simulink model "soccerbot"  (R2017b)
settings: Solver=FixedStepDiscrete  StartTime=0.0  StopTime=inf  FixedStep=0.01  RelTol=1e-3
PreLoadFcn:
  | clear;
  | 
  | % Sample times
  | sampleTime = 0.2;
  | 
  | % Control parameters
  | ctrlParam1 = 2;
  | ctrlParam2 = 3.5;
  | 
  | loadIpAddresses;
InitFcn:
  | loadFixedTrajectories;
model workspace (MAT data in the model file):
  SL_ROS_VariableLengthArrays_MaxSizes.CommonInfo.ArrayTruncateAction = 'EmitWarning'
  SL_ROS_VariableLengthArrays_MaxSizes.MsgTypeMap = containers.Map
  SL_ROS_VariableLengthArrays_MaxSizes.MsgTypeMap.serialization.keys = {'sensor_msgs/Image'}
  SL_ROS_VariableLengthArrays_MaxSizes.MsgTypeMap.serialization.values{1}(1).PropertyName = 'Data'
  SL_ROS_VariableLengthArrays_MaxSizes.MsgTypeMap.serialization.values{1}(1).DataType = 'uint8'
  SL_ROS_VariableLengthArrays_MaxSizes.MsgTypeMap.serialization.values{1}(1).MaxLength = 230400
  SL_ROS_VariableLengthArrays_MaxSizes.MsgTypeMap.serialization.values{1}(2).PropertyName = 'Encoding'
  SL_ROS_VariableLengthArrays_MaxSizes.MsgTypeMap.serialization.values{1}(2).DataType = 'uint8'
  SL_ROS_VariableLengthArrays_MaxSizes.MsgTypeMap.serialization.values{1}(2).MaxLength = 128
  SL_ROS_VariableLengthArrays_MaxSizes.MsgTypeMap.serialization.uniformity = 0
  SL_ROS_VariableLengthArrays_MaxSizes.MsgTypeMap.serialization.keyType = 'char'
  SL_ROS_VariableLengthArrays_MaxSizes.MsgTypeMap.serialization.valueType = 'any'
  ctrlParam1 = 1
  ctrlParam2 = 1.5
  sampleTime = 0.01
undefined symbols (not defined in the file): customState, getUpBackTraj, getUpFrontTraj, resting, walkTraj
libraries: simulink x54, robotlib x4, commblkintrlv2 x2, visionsinks x1
settings Model: Creator=scastro  LastModifiedBy=vuwij
settings OptimizationCC: PassReuseOutputArgsThreshold=0  EfficientMapNaN2IntZero=off  MaxStackSize=64
settings DebuggingCC: ParameterTunabilityLossMsg=error
settings HardwareCC: ProdBitPerPointer=32  ProdBitPerSizeT=32  ProdBitPerPtrDiffT=32  ProdLargestAtomicFloat=None  ProdIntDivRoundTo=Undefined  ProdEndianess=Unspecified  ProdWordSize=32  ProdHWDeviceType=Generic->Unspecified (assume 32-bit Generic)  TargetBitPerLong=64  TargetBitPerPointer=64  TargetBitPerSizeT=64  TargetBitPerPtrDiffT=64  TargetLongLongMode=on  TargetIntDivRoundTo=Zero  TargetEndianess=LittleEndian  TargetWordSize=64  TargetHWDeviceType=MATLAB Host  ProdEqTarget=off
settings SFSimCC: MATLABDynamicMemAlloc=off
settings RTWCC: TargetLang=C++
settings CodeAppCC: MaxIdLength=128
settings GRTTargetCC: TargetLangStandard=C89/C90 (ANSI)  CombineOutputUpdateFcns=off  GRTInterface=on

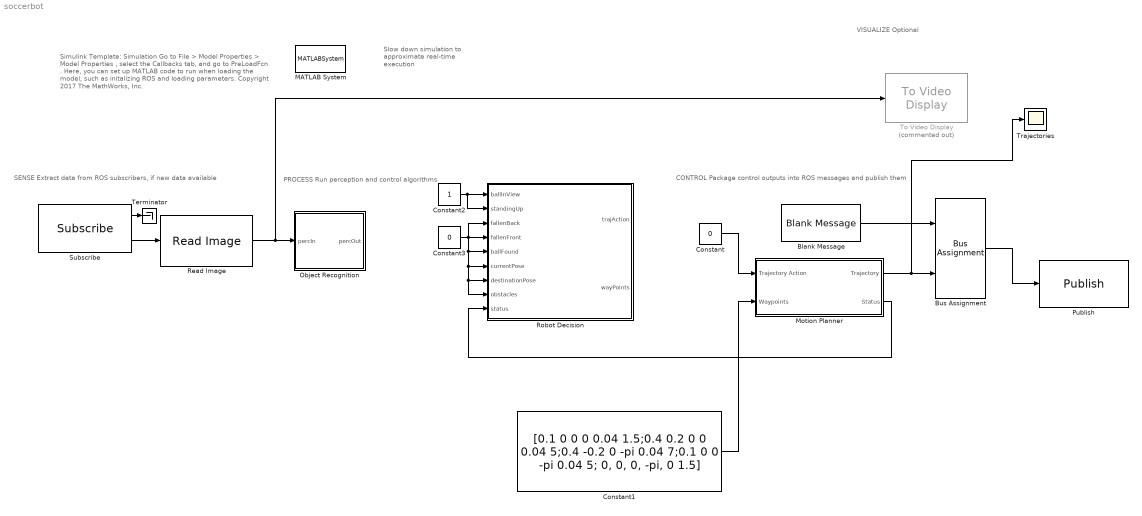
== system soccerbot ==
  note: Simulink Template: Simulation
      |
      | Go to File > Model Properties > Model Properties , select the Callbacks tab, and go to PreLoadFcn .
      |
      | Here, you can set up MATLAB code to run when loading the model, such as initalizing ROS and loading parameters.
      |
      | Copyright 2017 The MathWorks, Inc.
  note: Slow down simulation to approximate real-time execution
  note: PROCESS
      | Run perception and control algorithms
  note: SENSE
      | Extract data from ROS subscribers, if new data available
  note: VISUALIZE
      | Optional
  note: CONTROL
      | Package control outputs into ROS messages and publish them
  Blank Message : robotlib/Blank Message  SourceLibraryInfo=This block requires Robotics System Toolbox  messageType=soccer_msgs/RobotGoal  SampleTime=inf
      settings: SourceProductBaseCode=RO
  Bus Assignment : BusAssignment  AssignedSignals=Trajectories
  Constant : Constant  Value=0
  Constant1 : Constant  Value=[0.1 0 0 0 0.04 1.5;0.4 0.2 0 0 0.04 5;0.4 -0.2 0 -pi 0.04 7;0.1 0 0 -pi 0.04 5; 0, 0, 0, -pi, 0 1.5]  VectorParams1D=off
  Constant2 : Constant
  Constant3 : Constant  Value=0
  MATLAB System : MATLABSystem  System=ExampleHelperSimulationRateControl  SampleTime=sampleTime
      mask Type: ExampleHelperSimulationRateControl
      mask Display: disp('Rate Control');
  Motion Planner : Subsystem
  Object Recognition : Subsystem
  Publish : robotlib/Publish  SourceLibraryInfo=This block requires Robotics System Toolbox  topicSource=Select from ROS network  topic=/robotGoal  messageType=soccer_msgs/RobotGoal  messageQueueLength=1
      settings: SourceProductBaseCode=RO
  Read Image : robotlib/Read Image  SourceLibraryInfo=This block requires Robotics System Toolbox  MaximumImageSize=[240, 320]  ImageEncoding=rgb8  ShowAlphaOutput=off  ShowErrorCodeOutput=off  VariableSizeOutputs=off
      settings: SourceProductName=Robotics System Toolbox  SourceProductBaseCode=RO
  Robot Decision : Stateflow chart  TreatAsAtomicUnit=on
  Subscribe : robotlib/Subscribe  SourceLibraryInfo=This block requires Robotics System Toolbox  topicSource=Select from ROS network  topic=/soccerbot/camera1/image_raw  messageType=sensor_msgs/Image  sampleTime=-1  messageQueueLength=1
      settings: SourceProductBaseCode=RO
  Terminator : Terminator
  To Video Display : visionsinks/To Video Display  Commented=on  windowSizeMode=Normal  openAtMdlStart=on  fullScreen=off  videoWindowX=275  videoWindowY=548  saveWindowSize=off  videoWindowWidth=320  videoWindowHeight=240  inputColorFormat=RGB  inputType=Obsolete  imagePorts=One multidimensional signal  OutputDevice=On-screen video monitor  dataOrg=Column-major  isWindowOpen=off
      settings: SourceProductName=Computer Vision System Toolbox
  Trajectories : Scope
  wires:
  Read Image/1 -> To Video Display/1, Object Recognition/1(percIn)
  Subscribe/2 -> Read Image/1
  Subscribe/1 -> Terminator/1
  Motion Planner/1(Trajectory) -> Trajectories/1, Bus Assignment/2
  Bus Assignment/1 -> Publish/1
  Blank Message/1 -> Bus Assignment/1
  Constant1/1 -> Motion Planner/2(Waypoints)
  Constant/1 -> Motion Planner/1(Trajectory Action)
  Constant2/1 -> Robot Decision/2(standingUp), Robot Decision/1(ballInView)
  Constant3/1 -> Robot Decision/3(fallenBack), Robot Decision/8(obstacles), Robot Decision/7(destinationPose), Robot Decision/6(currentPose), Robot Decision/5(ballFound), Robot Decision/4(fallenFront)
  Motion Planner/2(Status) -> Robot Decision/9(status)

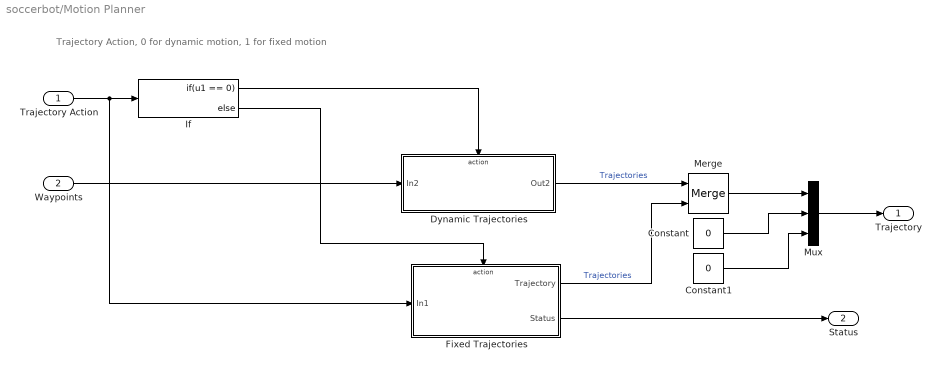
== system soccerbot/Motion Planner ==
  note: Trajectory Action, 0 for dynamic motion, 1 for fixed motion
  Trajectory Action : Inport
  Waypoints : Inport  Port=2
  Constant : Constant  Value=0  OutDataTypeStr=single
  Constant1 : Constant  Value=0  OutDataTypeStr=single
  Dynamic Trajectories : Subsystem  TreatAsAtomicUnit=on
  Fixed Trajectories : Subsystem  TreatAsAtomicUnit=on
  If : If  IfExpression=u1 == 0
  Merge : Merge
  Mux : Mux  Inputs=3
  Trajectory : Outport
  Status : Outport  Port=2
  wires:
  Dynamic Trajectories/1(Out2) -> Merge/1  "Trajectories"
  If/1 -> Dynamic Trajectories/Action
  Trajectory Action/1 -> Fixed Trajectories/1(In1), If/1
  Fixed Trajectories/1(Trajectory) -> Merge/2  "Trajectories"
  If/2 -> Fixed Trajectories/Action
  Waypoints/1 -> Dynamic Trajectories/1(In2)
  Fixed Trajectories/2(Status) -> Status/1
  Merge/1 -> Mux/1
  Mux/1 -> Trajectory/1
  Constant/1 -> Mux/2
  Constant1/1 -> Mux/3

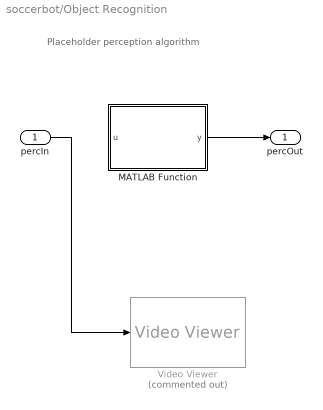
== system soccerbot/Object Recognition ==
  note: Placeholder perception algorithm
  percIn : Inport
  MATLAB Function : MATLAB Function  TreatAsAtomicUnit=on
  Video Viewer : VideoViewer  Commented=on  FigPos=[511 723 604 426]
  percOut : Outport
  wires:
  percIn/1 -> Video Viewer/1
  MATLAB Function/1(y) -> percOut/1

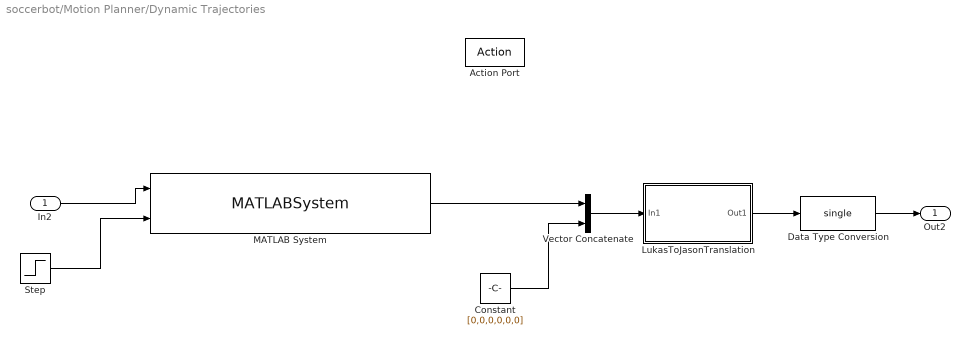
== system soccerbot/Motion Planner/Dynamic Trajectories ==
  In2 : Inport
  Action Port : ActionPort  ActionType=then
  Constant : Constant  Value=[0,0,0,0,0,0]
  Data Type Conversion : DataTypeConversion  OutDataTypeStr=single
  LukasToJasonTranslation : Subsystem  TreatAsAtomicUnit=on
  MATLAB System : MATLABSystem  System=BipedalRobotSystemObject  SimulateUsing=Interpreted execution
      mask Type: BipedalRobotSystemObject
      mask Display:
      | disp('BipedalRobotSystemObject');
      | port_label('input',1,'waypoints');
      | port_label('input',2,'trigger');
      | port_label('output',1,'trajectories');
  Step : Step  Time=3  SampleTime=0
  Vector Concatenate : Concatenate
  Out2 : Outport
  wires:
  In2/1 -> MATLAB System/1
  Constant/1 -> Vector Concatenate/2
  Vector Concatenate/1 -> LukasToJasonTranslation/1(In1)
  Step/1 -> MATLAB System/2
  MATLAB System/1 -> Vector Concatenate/1
  LukasToJasonTranslation/1(Out1) -> Data Type Conversion/1
  Data Type Conversion/1 -> Out2/1

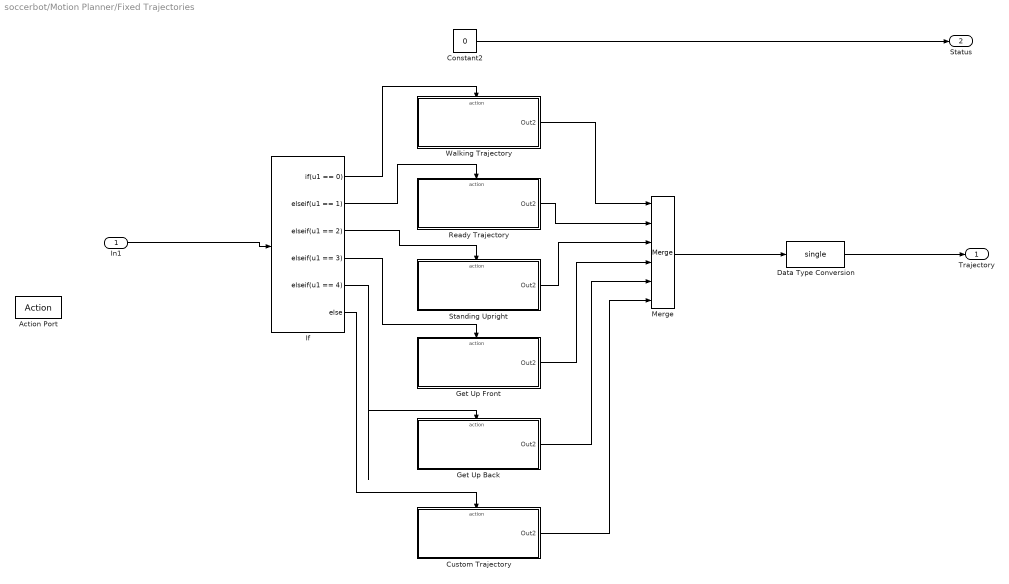
== system soccerbot/Motion Planner/Fixed Trajectories ==
  In1 : Inport
  Action Port : ActionPort  ActionType=else
  Constant2 : Constant  Value=0
  "Custom Trajectory " : Subsystem  TreatAsAtomicUnit=on
  Data Type Conversion : DataTypeConversion  OutDataTypeStr=single
  Get Up Back : Subsystem  TreatAsAtomicUnit=on
  Get Up Front : Subsystem  TreatAsAtomicUnit=on
  If : If  IfExpression=u1 == 0  ElseIfExpressions=u1 == 1, u1 == 2, u1 == 3, u1 == 4
  Merge : Merge  Inputs=6
  Ready Trajectory : Subsystem  TreatAsAtomicUnit=on
  Standing Upright : Subsystem  TreatAsAtomicUnit=on
  Walking Trajectory : Subsystem  TreatAsAtomicUnit=on
  Trajectory : Outport
  Status : Outport  Port=2
  wires:
  Standing Upright/1(Out2) -> Merge/3
  Get Up Back/1(Out2) -> Merge/5
  If/4 -> Get Up Front/Action
  If/1 -> Walking Trajectory/Action
  Walking Trajectory/1(Out2) -> Merge/1
  Data Type Conversion/1 -> Trajectory/1
  Ready Trajectory/1(Out2) -> Merge/2
  Merge/1 -> Data Type Conversion/1
  If/6 -> "Custom Trajectory "/Action
  In1/1 -> If/1
  "Custom Trajectory "/1(Out2) -> Merge/6
  If/5 -> Get Up Back/Action
  If/3 -> Standing Upright/Action
  Constant2/1 -> Status/1
  Get Up Front/1(Out2) -> Merge/4
  If/2 -> Ready Trajectory/Action

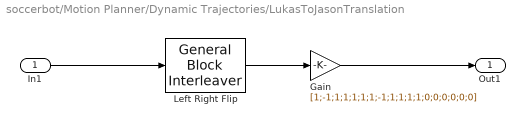
== system soccerbot/Motion Planner/Dynamic Trajectories/LukasToJasonTranslation ==
  In1 : Inport
  Gain : Gain  Gain=[1;-1;1;1;1;1;1;-1;1;1;1;1;0;0;0;0;0;0]
  Left Right Flip : commblkintrlv2/General Block Interleaver  permutationVectorSource=Dialog  elements=[7;8;9;10;11;12;1;2;3;4;5;6;13;14;15;16;17;18]
      settings: SourceProductName=Communications System Toolbox  SourceProductBaseCode=CM
  Out1 : Outport
  wires:
  In1/1 -> Left Right Flip/1
  Gain/1 -> Out1/1
  Left Right Flip/1 -> Gain/1

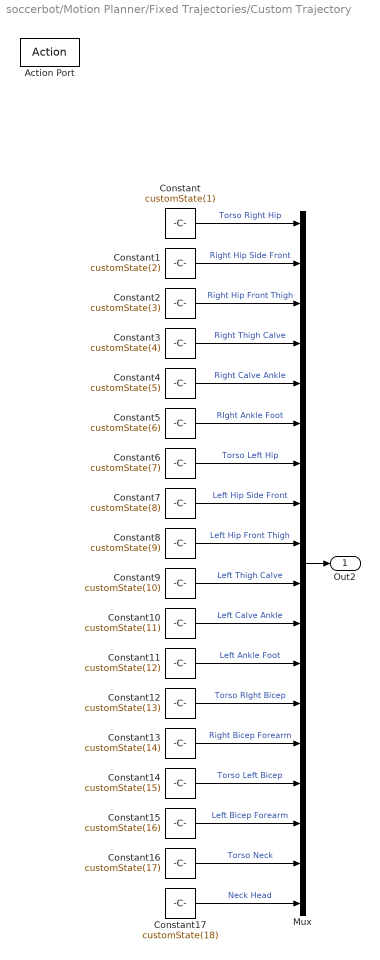
== system soccerbot/Motion Planner/Fixed Trajectories/Custom Trajectory  ==
  Action Port : ActionPort  ActionType=else
  Constant : Constant  Value=customState(1)
  Constant1 : Constant  Value=customState(2)
  Constant10 : Constant  Value=customState(11)
  Constant11 : Constant  Value=customState(12)
  Constant12 : Constant  Value=customState(13)
  Constant13 : Constant  Value=customState(14)
  Constant14 : Constant  Value=customState(15)
  Constant15 : Constant  Value=customState(16)
  Constant16 : Constant  Value=customState(17)
  Constant17 : Constant  Value=customState(18)
  Constant2 : Constant  Value=customState(3)
  Constant3 : Constant  Value=customState(4)
  Constant4 : Constant  Value=customState(5)
  Constant5 : Constant  Value=customState(6)
  Constant6 : Constant  Value=customState(7)
  Constant7 : Constant  Value=customState(8)
  Constant8 : Constant  Value=customState(9)
  Constant9 : Constant  Value=customState(10)
  Mux : Mux  Inputs=18
  Out2 : Outport
  wires:
  Constant3/1 -> Mux/4  "Right Thigh Calve"
  Constant12/1 -> Mux/13  "Torso RIght Bicep"
  Constant8/1 -> Mux/9  "Left Hip Front Thigh"
  Constant1/1 -> Mux/2  "Right Hip Side Front"
  Constant14/1 -> Mux/15  "Torso Left Bicep"
  Constant9/1 -> Mux/10  "Left Thigh Calve"
  Constant17/1 -> Mux/18  "Neck Head"
  Constant11/1 -> Mux/12  "Left Ankle Foot"
  Constant16/1 -> Mux/17  "Torso Neck"
  Constant10/1 -> Mux/11  "Left Calve Ankle"
  Constant15/1 -> Mux/16  "Left Bicep Forearm"
  Constant13/1 -> Mux/14  "Right Bicep Forearm"
  Constant/1 -> Mux/1  "Torso Right Hip"
  Mux/1 -> Out2/1
  Constant7/1 -> Mux/8  "Left Hip Side Front"
  Constant2/1 -> Mux/3  "Right Hip Front Thigh"
  Constant6/1 -> Mux/7  "Torso Left Hip"
  Constant4/1 -> Mux/5  "Right Calve Ankle"
  Constant5/1 -> Mux/6  "RIght Ankle Foot"

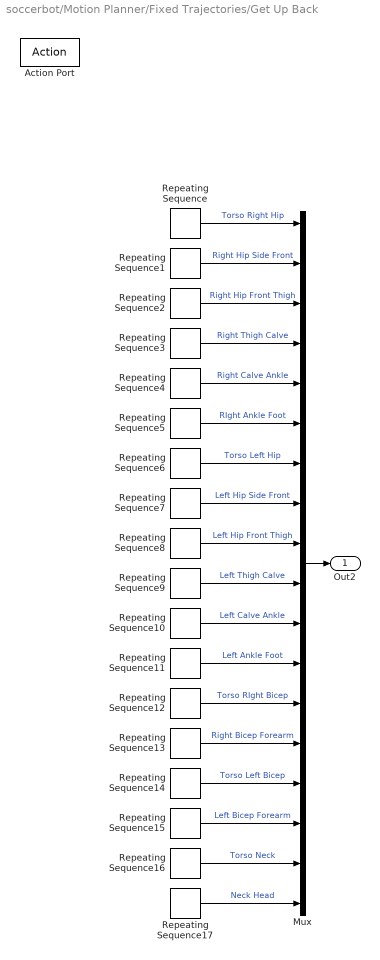
== system soccerbot/Motion Planner/Fixed Trajectories/Get Up Back ==
  Action Port : ActionPort  ActionType=elseif
  Mux : Mux  Inputs=18
  Repeating Sequence : simulink/Sources/Repeating Sequence  rep_seq_t=getUpBackTrajTime  rep_seq_y=getUpBackTraj(:,1)
  Repeating Sequence1 : simulink/Sources/Repeating Sequence  rep_seq_t=getUpBackTrajTime  rep_seq_y=getUpBackTraj(:,2)
  Repeating Sequence10 : simulink/Sources/Repeating Sequence  rep_seq_t=getUpBackTrajTime  rep_seq_y=getUpBackTraj(:,11)
  Repeating Sequence11 : simulink/Sources/Repeating Sequence  rep_seq_t=getUpBackTrajTime  rep_seq_y=getUpBackTraj(:,12)
  Repeating Sequence12 : simulink/Sources/Repeating Sequence  rep_seq_t=getUpBackTrajTime  rep_seq_y=getUpBackTraj(:,13)
  Repeating Sequence13 : simulink/Sources/Repeating Sequence  rep_seq_t=getUpBackTrajTime  rep_seq_y=getUpBackTraj(:,14)
  Repeating Sequence14 : simulink/Sources/Repeating Sequence  rep_seq_t=getUpBackTrajTime  rep_seq_y=getUpBackTraj(:,15)
  Repeating Sequence15 : simulink/Sources/Repeating Sequence  rep_seq_t=getUpBackTrajTime  rep_seq_y=getUpBackTraj(:,16)
  Repeating Sequence16 : simulink/Sources/Repeating Sequence  rep_seq_t=getUpBackTrajTime  rep_seq_y=getUpBackTraj(:,17)
  Repeating Sequence17 : simulink/Sources/Repeating Sequence  rep_seq_t=getUpBackTrajTime  rep_seq_y=getUpBackTraj(:,18)
  Repeating Sequence2 : simulink/Sources/Repeating Sequence  rep_seq_t=getUpBackTrajTime  rep_seq_y=getUpBackTraj(:,3)
  Repeating Sequence3 : simulink/Sources/Repeating Sequence  rep_seq_t=getUpBackTrajTime  rep_seq_y=getUpBackTraj(:,4)
  Repeating Sequence4 : simulink/Sources/Repeating Sequence  rep_seq_t=getUpBackTrajTime  rep_seq_y=getUpBackTraj(:,5)
  Repeating Sequence5 : simulink/Sources/Repeating Sequence  rep_seq_t=getUpBackTrajTime  rep_seq_y=getUpBackTraj(:,6)
  Repeating Sequence6 : simulink/Sources/Repeating Sequence  rep_seq_t=getUpBackTrajTime  rep_seq_y=getUpBackTraj(:,6)
  Repeating Sequence7 : simulink/Sources/Repeating Sequence  rep_seq_t=getUpBackTrajTime  rep_seq_y=getUpBackTraj(:,8)
  Repeating Sequence8 : simulink/Sources/Repeating Sequence  rep_seq_t=getUpBackTrajTime  rep_seq_y=getUpBackTraj(:,9)
  Repeating Sequence9 : simulink/Sources/Repeating Sequence  rep_seq_t=getUpBackTrajTime  rep_seq_y=getUpBackTraj(:,10)
  Out2 : Outport
  wires:
  Repeating Sequence3/1 -> Mux/4  "Right Thigh Calve"
  Repeating Sequence12/1 -> Mux/13  "Torso RIght Bicep"
  Repeating Sequence8/1 -> Mux/9  "Left Hip Front Thigh"
  Repeating Sequence1/1 -> Mux/2  "Right Hip Side Front"
  Repeating Sequence14/1 -> Mux/15  "Torso Left Bicep"
  Repeating Sequence9/1 -> Mux/10  "Left Thigh Calve"
  Repeating Sequence17/1 -> Mux/18  "Neck Head"
  Repeating Sequence11/1 -> Mux/12  "Left Ankle Foot"
  Repeating Sequence16/1 -> Mux/17  "Torso Neck"
  Repeating Sequence10/1 -> Mux/11  "Left Calve Ankle"
  Repeating Sequence15/1 -> Mux/16  "Left Bicep Forearm"
  Repeating Sequence13/1 -> Mux/14  "Right Bicep Forearm"
  Repeating Sequence/1 -> Mux/1  "Torso Right Hip"
  Mux/1 -> Out2/1
  Repeating Sequence7/1 -> Mux/8  "Left Hip Side Front"
  Repeating Sequence2/1 -> Mux/3  "Right Hip Front Thigh"
  Repeating Sequence6/1 -> Mux/7  "Torso Left Hip"
  Repeating Sequence4/1 -> Mux/5  "Right Calve Ankle"
  Repeating Sequence5/1 -> Mux/6  "RIght Ankle Foot"

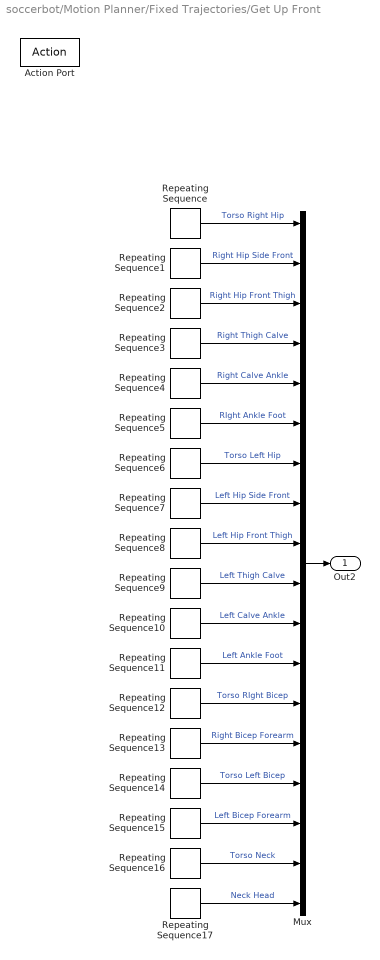
== system soccerbot/Motion Planner/Fixed Trajectories/Get Up Front ==
  Action Port : ActionPort  ActionType=elseif
  Mux : Mux  Inputs=18
  Repeating Sequence : simulink/Sources/Repeating Sequence  rep_seq_t=getUpFrontTrajTime  rep_seq_y=getUpFrontTraj(:,1)
  Repeating Sequence1 : simulink/Sources/Repeating Sequence  rep_seq_t=getUpFrontTrajTime  rep_seq_y=getUpFrontTraj(:,2)
  Repeating Sequence10 : simulink/Sources/Repeating Sequence  rep_seq_t=getUpFrontTrajTime  rep_seq_y=getUpFrontTraj(:,11)
  Repeating Sequence11 : simulink/Sources/Repeating Sequence  rep_seq_t=getUpFrontTrajTime  rep_seq_y=getUpFrontTraj(:,12)
  Repeating Sequence12 : simulink/Sources/Repeating Sequence  rep_seq_t=getUpFrontTrajTime  rep_seq_y=getUpFrontTraj(:,13)
  Repeating Sequence13 : simulink/Sources/Repeating Sequence  rep_seq_t=getUpFrontTrajTime  rep_seq_y=getUpFrontTraj(:,14)
  Repeating Sequence14 : simulink/Sources/Repeating Sequence  rep_seq_t=getUpFrontTrajTime  rep_seq_y=getUpFrontTraj(:,15)
  Repeating Sequence15 : simulink/Sources/Repeating Sequence  rep_seq_t=getUpFrontTrajTime  rep_seq_y=getUpFrontTraj(:,16)
  Repeating Sequence16 : simulink/Sources/Repeating Sequence  rep_seq_t=getUpFrontTrajTime  rep_seq_y=getUpFrontTraj(:,17)
  Repeating Sequence17 : simulink/Sources/Repeating Sequence  rep_seq_t=getUpFrontTrajTime  rep_seq_y=getUpFrontTraj(:,18)
  Repeating Sequence2 : simulink/Sources/Repeating Sequence  rep_seq_t=getUpFrontTrajTime  rep_seq_y=getUpFrontTraj(:,3)
  Repeating Sequence3 : simulink/Sources/Repeating Sequence  rep_seq_t=getUpFrontTrajTime  rep_seq_y=getUpFrontTraj(:,4)
  Repeating Sequence4 : simulink/Sources/Repeating Sequence  rep_seq_t=getUpFrontTrajTime  rep_seq_y=getUpFrontTraj(:,5)
  Repeating Sequence5 : simulink/Sources/Repeating Sequence  rep_seq_t=getUpFrontTrajTime  rep_seq_y=getUpFrontTraj(:,6)
  Repeating Sequence6 : simulink/Sources/Repeating Sequence  rep_seq_t=getUpFrontTrajTime  rep_seq_y=getUpFrontTraj(:,7)
  Repeating Sequence7 : simulink/Sources/Repeating Sequence  rep_seq_t=getUpFrontTrajTime  rep_seq_y=getUpFrontTraj(:,8)
  Repeating Sequence8 : simulink/Sources/Repeating Sequence  rep_seq_t=getUpFrontTrajTime  rep_seq_y=getUpFrontTraj(:,9)
  Repeating Sequence9 : simulink/Sources/Repeating Sequence  rep_seq_t=getUpFrontTrajTime  rep_seq_y=getUpFrontTraj(:,10)
  Out2 : Outport
  wires:
  Repeating Sequence3/1 -> Mux/4  "Right Thigh Calve"
  Repeating Sequence12/1 -> Mux/13  "Torso RIght Bicep"
  Repeating Sequence8/1 -> Mux/9  "Left Hip Front Thigh"
  Repeating Sequence1/1 -> Mux/2  "Right Hip Side Front"
  Repeating Sequence14/1 -> Mux/15  "Torso Left Bicep"
  Repeating Sequence9/1 -> Mux/10  "Left Thigh Calve"
  Repeating Sequence17/1 -> Mux/18  "Neck Head"
  Repeating Sequence11/1 -> Mux/12  "Left Ankle Foot"
  Repeating Sequence16/1 -> Mux/17  "Torso Neck"
  Repeating Sequence10/1 -> Mux/11  "Left Calve Ankle"
  Repeating Sequence15/1 -> Mux/16  "Left Bicep Forearm"
  Repeating Sequence13/1 -> Mux/14  "Right Bicep Forearm"
  Repeating Sequence/1 -> Mux/1  "Torso Right Hip"
  Mux/1 -> Out2/1
  Repeating Sequence7/1 -> Mux/8  "Left Hip Side Front"
  Repeating Sequence2/1 -> Mux/3  "Right Hip Front Thigh"
  Repeating Sequence6/1 -> Mux/7  "Torso Left Hip"
  Repeating Sequence4/1 -> Mux/5  "Right Calve Ankle"
  Repeating Sequence5/1 -> Mux/6  "RIght Ankle Foot"

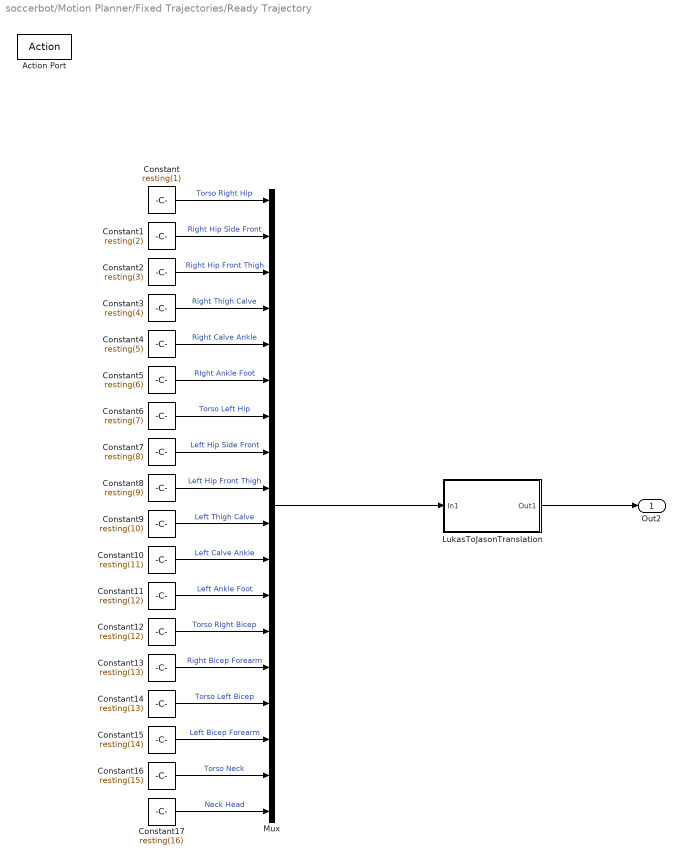
== system soccerbot/Motion Planner/Fixed Trajectories/Ready Trajectory ==
  Action Port : ActionPort  ActionType=elseif
  Constant : Constant  Value=resting(1)
  Constant1 : Constant  Value=resting(2)
  Constant10 : Constant  Value=resting(11)
  Constant11 : Constant  Value=resting(12)
  Constant12 : Constant  Value=resting(12)
  Constant13 : Constant  Value=resting(13)
  Constant14 : Constant  Value=resting(13)
  Constant15 : Constant  Value=resting(14)
  Constant16 : Constant  Value=resting(15)
  Constant17 : Constant  Value=resting(16)
  Constant2 : Constant  Value=resting(3)
  Constant3 : Constant  Value=resting(4)
  Constant4 : Constant  Value=resting(5)
  Constant5 : Constant  Value=resting(6)
  Constant6 : Constant  Value=resting(7)
  Constant7 : Constant  Value=resting(8)
  Constant8 : Constant  Value=resting(9)
  Constant9 : Constant  Value=resting(10)
  LukasToJasonTranslation : Subsystem
  Mux : Mux  Inputs=18
  Out2 : Outport
  wires:
  Constant3/1 -> Mux/4  "Right Thigh Calve"
  Constant12/1 -> Mux/13  "Torso RIght Bicep"
  Constant8/1 -> Mux/9  "Left Hip Front Thigh"
  Constant1/1 -> Mux/2  "Right Hip Side Front"
  Constant14/1 -> Mux/15  "Torso Left Bicep"
  Constant9/1 -> Mux/10  "Left Thigh Calve"
  Constant17/1 -> Mux/18  "Neck Head"
  Constant11/1 -> Mux/12  "Left Ankle Foot"
  Constant16/1 -> Mux/17  "Torso Neck"
  Constant10/1 -> Mux/11  "Left Calve Ankle"
  Constant15/1 -> Mux/16  "Left Bicep Forearm"
  Constant13/1 -> Mux/14  "Right Bicep Forearm"
  Constant/1 -> Mux/1  "Torso Right Hip"
  Constant7/1 -> Mux/8  "Left Hip Side Front"
  Constant2/1 -> Mux/3  "Right Hip Front Thigh"
  Constant6/1 -> Mux/7  "Torso Left Hip"
  Constant4/1 -> Mux/5  "Right Calve Ankle"
  Constant5/1 -> Mux/6  "RIght Ankle Foot"
  Mux/1 -> LukasToJasonTranslation/1(In1)
  LukasToJasonTranslation/1(Out1) -> Out2/1

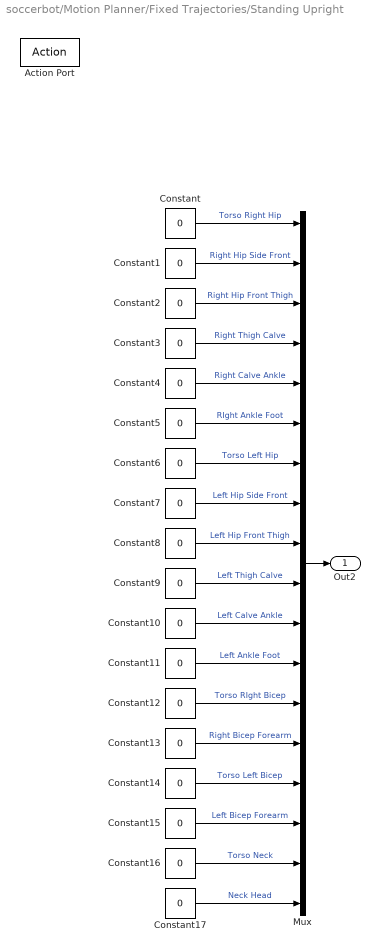
== system soccerbot/Motion Planner/Fixed Trajectories/Standing Upright ==
  Action Port : ActionPort  ActionType=elseif
  Constant{,1..17} (18 alike) : Constant  Value=0
  Mux : Mux  Inputs=18
  Out2 : Outport
  wires:
  Constant3/1 -> Mux/4  "Right Thigh Calve"
  Constant12/1 -> Mux/13  "Torso RIght Bicep"
  Constant8/1 -> Mux/9  "Left Hip Front Thigh"
  Constant1/1 -> Mux/2  "Right Hip Side Front"
  Constant14/1 -> Mux/15  "Torso Left Bicep"
  Constant9/1 -> Mux/10  "Left Thigh Calve"
  Constant17/1 -> Mux/18  "Neck Head"
  Constant11/1 -> Mux/12  "Left Ankle Foot"
  Constant16/1 -> Mux/17  "Torso Neck"
  Constant10/1 -> Mux/11  "Left Calve Ankle"
  Constant15/1 -> Mux/16  "Left Bicep Forearm"
  Constant13/1 -> Mux/14  "Right Bicep Forearm"
  Constant/1 -> Mux/1  "Torso Right Hip"
  Mux/1 -> Out2/1
  Constant7/1 -> Mux/8  "Left Hip Side Front"
  Constant2/1 -> Mux/3  "Right Hip Front Thigh"
  Constant6/1 -> Mux/7  "Torso Left Hip"
  Constant4/1 -> Mux/5  "Right Calve Ankle"
  Constant5/1 -> Mux/6  "RIght Ankle Foot"

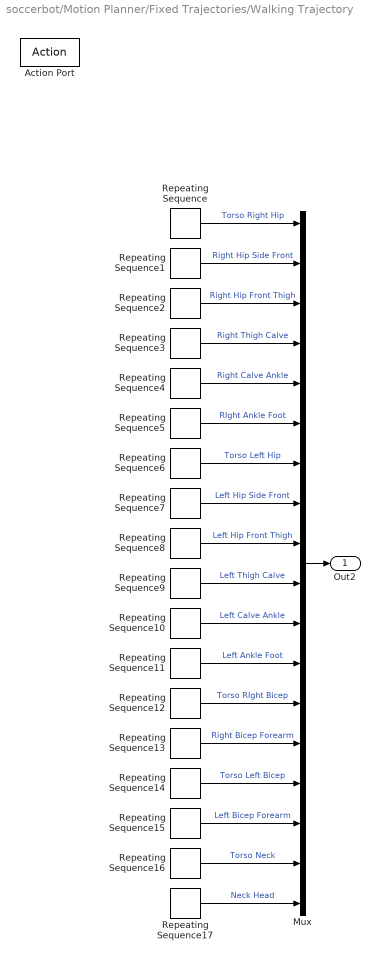
== system soccerbot/Motion Planner/Fixed Trajectories/Walking Trajectory ==
  Action Port : ActionPort  ActionType=then
  Mux : Mux  Inputs=18
  Repeating Sequence : simulink/Sources/Repeating Sequence  rep_seq_t=walkTrajTime  rep_seq_y=walkTraj(:,1)
  Repeating Sequence1 : simulink/Sources/Repeating Sequence  rep_seq_t=walkTrajTime  rep_seq_y=walkTraj(:,2)
  Repeating Sequence10 : simulink/Sources/Repeating Sequence  rep_seq_t=walkTrajTime  rep_seq_y=walkTraj(:,11)
  Repeating Sequence11 : simulink/Sources/Repeating Sequence  rep_seq_t=walkTrajTime  rep_seq_y=walkTraj(:,12)
  Repeating Sequence12 : simulink/Sources/Repeating Sequence  rep_seq_t=walkTrajTime  rep_seq_y=walkTraj(:,13)
  Repeating Sequence13 : simulink/Sources/Repeating Sequence  rep_seq_t=walkTrajTime  rep_seq_y=walkTraj(:,14)
  Repeating Sequence14 : simulink/Sources/Repeating Sequence  rep_seq_t=walkTrajTime  rep_seq_y=walkTraj(:,15)
  Repeating Sequence15 : simulink/Sources/Repeating Sequence  rep_seq_t=walkTrajTime  rep_seq_y=walkTraj(:,16)
  Repeating Sequence16 : simulink/Sources/Repeating Sequence  rep_seq_t=walkTrajTime  rep_seq_y=walkTraj(:,17)
  Repeating Sequence17 : simulink/Sources/Repeating Sequence  rep_seq_t=walkTrajTime  rep_seq_y=walkTraj(:,18)
  Repeating Sequence2 : simulink/Sources/Repeating Sequence  rep_seq_t=walkTrajTime  rep_seq_y=walkTraj(:,3)
  Repeating Sequence3 : simulink/Sources/Repeating Sequence  rep_seq_t=walkTrajTime  rep_seq_y=walkTraj(:,4)
  Repeating Sequence4 : simulink/Sources/Repeating Sequence  rep_seq_t=walkTrajTime  rep_seq_y=walkTraj(:,5)
  Repeating Sequence5 : simulink/Sources/Repeating Sequence  rep_seq_t=walkTrajTime  rep_seq_y=walkTraj(:,6)
  Repeating Sequence6 : simulink/Sources/Repeating Sequence  rep_seq_t=walkTrajTime  rep_seq_y=walkTraj(:,7)
  Repeating Sequence7 : simulink/Sources/Repeating Sequence  rep_seq_t=walkTrajTime  rep_seq_y=walkTraj(:,8)
  Repeating Sequence8 : simulink/Sources/Repeating Sequence  rep_seq_t=walkTrajTime  rep_seq_y=walkTraj(:,9)
  Repeating Sequence9 : simulink/Sources/Repeating Sequence  rep_seq_t=walkTrajTime  rep_seq_y=walkTraj(:,10)
  Out2 : Outport
  wires:
  Repeating Sequence3/1 -> Mux/4  "Right Thigh Calve"
  Repeating Sequence12/1 -> Mux/13  "Torso RIght Bicep"
  Repeating Sequence8/1 -> Mux/9  "Left Hip Front Thigh"
  Repeating Sequence1/1 -> Mux/2  "Right Hip Side Front"
  Repeating Sequence14/1 -> Mux/15  "Torso Left Bicep"
  Repeating Sequence9/1 -> Mux/10  "Left Thigh Calve"
  Repeating Sequence17/1 -> Mux/18  "Neck Head"
  Repeating Sequence11/1 -> Mux/12  "Left Ankle Foot"
  Repeating Sequence16/1 -> Mux/17  "Torso Neck"
  Repeating Sequence10/1 -> Mux/11  "Left Calve Ankle"
  Repeating Sequence15/1 -> Mux/16  "Left Bicep Forearm"
  Repeating Sequence13/1 -> Mux/14  "Right Bicep Forearm"
  Repeating Sequence/1 -> Mux/1  "Torso Right Hip"
  Mux/1 -> Out2/1
  Repeating Sequence7/1 -> Mux/8  "Left Hip Side Front"
  Repeating Sequence2/1 -> Mux/3  "Right Hip Front Thigh"
  Repeating Sequence6/1 -> Mux/7  "Torso Left Hip"
  Repeating Sequence4/1 -> Mux/5  "Right Calve Ankle"
  Repeating Sequence5/1 -> Mux/6  "RIght Ankle Foot"

== system soccerbot/Motion Planner/Fixed Trajectories/Ready Trajectory/LukasToJasonTranslation ==
  In1 : Inport
  Gain : Gain  Gain=[-1;-1;-1;-1;-1;-1;-1;-1;-1;-1;-1;-1;0;0;0;0;0;0]
  Left Right Flip : commblkintrlv2/General Block Interleaver  permutationVectorSource=Dialog  elements=[7;8;9;10;11;12;1;2;3;4;5;6;13;14;15;16;17;18]
      settings: SourceProductName=Communications System Toolbox  SourceProductBaseCode=CM
  Out1 : Outport
  wires:
  In1/1 -> Left Right Flip/1
  Gain/1 -> Out1/1
  Left Right Flip/1 -> Gain/1

== matlab function soccerbot/Object Recognition/MATLAB Function ==
  data: u input; y output
function y = myPerceptionFcn(u)

y = 2*u;

== stateflow chart soccerbot/Robot Decision ==
  state SearchForBall
  state FallenFront
    entry: trajAction = 3;
  state Idle
    entry: trajAction = 6
  state Walking
    entry: trajAction = 0;
    wayPoints = findWayPoints(currentPose, obstacles, destinationPose);
  state FallenBack
  FallenFront -> Idle [order 1] : [status == 1 && fallenBack ~= 1 && fallenFront ~= 1]
  SearchForBall -> SearchForBall [order 1] : [status==1 && ballFound==0]
  FallenFront -> FallenFront [order 3] : [status == 1 && fallenFront == 1]
  (default) -> Idle
  Idle -> SearchForBall : [ fallenBack ~= 1 && fallenFront ~= 1 && after(3,sec)]
  SearchForBall -> FallenFront [order 2] : [fallenFront == 1]
  SearchForBall -> FallenBack [order 3] : [fallenBack == 1]
  Walking -> FallenFront [order 1] : [fallenFront == 1]
  SearchForBall -> Walking [order 4] : [status==1 && ballFound == 1]
  FallenFront -> FallenBack [order 2] : [status == 1 && fallenBack == 1]
  FallenBack -> FallenFront [order 2] : [status == 1 && fallenFront == 1]
  Walking -> FallenBack [order 2] : [fallenBack == 1]
  FallenBack -> FallenBack [order 1] : [status == 1 && fallenBack== 1]
  data: curPose function_input; obs function_input; destPos function_input; waypoints function_output; ballInView input; standingUp input; fallenBack input; fallenFront input; ballFound input; currentPose input; destinationPose input; obstacles input; status input; trajAction output; wayPoints output
  function waypoints = findWayPoints(curPose, obs, destPos):
    | function waypoints = findWayPoints(curPose, obs, destPos)
    |     
    |     % Hardcoded poses
    |     pose2 = [0.1, 0, 0, 0, 0.04];
    |     pose3 = [0.4, 0.2, 0, 0, 0.04];
    |     pose4 = [0.4, -0.2, 0, -pi, 0.04];
    |     pose5 = [0.1, 0, 0, -pi, 0.04];
    |     pose6 = [0, 0, 0, -pi, 0.0];
    |     
    |     waypoints = [pose2, pose3, pose4, pose5, pose6];
    | end
